simulink model "Xango_car_metamodel_V1_funcional"  (R2015a)
settings: Solver=ode45  StartTime=0  StopTime=6  FixedStep=1e-3  MaxStep=0.0001  RelTol=1e-19
values from neighbouring files (symbols this model uses):
  B_x_dd = C_s_dd / (C_x * D_dd)    [Xango_car_metamodel_SCRIPT.m]
  B_x_de = C_s_de / (C_x * D_de)    [Xango_car_metamodel_SCRIPT.m]
  B_x_td = C_s_td / (C_x * D_td)    [Xango_car_metamodel_SCRIPT.m]
  B_x_te = C_s_te / (C_x * D_te)    [Xango_car_metamodel_SCRIPT.m]
  B_y_dd = C_s_dd / (C_y * D_dd)    [Xango_car_metamodel_SCRIPT.m]
  B_y_de = C_s_de / (C_y * D_de)    [Xango_car_metamodel_SCRIPT.m]
  B_y_td = C_s_td / (C_y * D_td)    [Xango_car_metamodel_SCRIPT.m]
  B_y_te = C_s_te / (C_y * D_te)    [Xango_car_metamodel_SCRIPT.m]
  C_alpha_d = 0.5    [Xango_car_metamodel_SCRIPT.m]
  C_alpha_e = 0.5    [Xango_car_metamodel_SCRIPT.m]
  C_x = 1.0    (= 1)    [Xango_car_metamodel_SCRIPT.m]
  C_y = 1.627    [Xango_car_metamodel_SCRIPT.m]
  Cdd = 3e3    (= 3000)    [Xango_car_metamodel_SCRIPT.m]
  Cde = 3e3    (= 3000)    [Xango_car_metamodel_SCRIPT.m]
  Ctd = 5e3    (= 5000)    [Xango_car_metamodel_SCRIPT.m]
  Cte = 5e3    (= 5000)    [Xango_car_metamodel_SCRIPT.m]
  D_dd = mu * F_zdd    (= 1066.8375)    [Xango_car_metamodel_SCRIPT.m]
  D_de = mu * F_zde    (= 1066.8375)    [Xango_car_metamodel_SCRIPT.m]
  D_td = mu * F_ztd    (= 1066.8375)    [Xango_car_metamodel_SCRIPT.m]
  D_te = mu * F_zte    (= 1066.8375)    [Xango_car_metamodel_SCRIPT.m]
  E = 0.3336564873588197    (= 0.333656487359)    [Xango_car_metamodel_SCRIPT.m]
  H_cg = 0.3    [Xango_car_metamodel_SCRIPT.m]
  I_beta = 1e7    (= 10000000)    [Xango_car_metamodel_SCRIPT.m]
  I_p = 1.0    (= 1)    [Xango_car_metamodel_SCRIPT.m]
  I_psi = 1e7    (= 10000000)    [Xango_car_metamodel_SCRIPT.m]
  I_rho = 1e7    (= 10000000)    [Xango_car_metamodel_SCRIPT.m]
  If = 5e6    (= 5000000)    [Xango_car_metamodel_SCRIPT.m]
  It = 5e6    (= 5000000)    [Xango_car_metamodel_SCRIPT.m]
  Kdd = 3e6    (= 3000000)    [Xango_car_metamodel_SCRIPT.m]
  Kde = 3e6    (= 3000000)    [Xango_car_metamodel_SCRIPT.m]
  Kf = 3.01e7    (= 30100000)    [Xango_car_metamodel_SCRIPT.m]
  Kpdd = 2e6    (= 2000000)    [Xango_car_metamodel_SCRIPT.m]
  Kpde = 2e6    (= 2000000)    [Xango_car_metamodel_SCRIPT.m]
  Kptd = 2e6    (= 2000000)    [Xango_car_metamodel_SCRIPT.m]
  Kpte = 2e6    (= 2000000)    [Xango_car_metamodel_SCRIPT.m]
  Kt = 1.6e7    (= 16000000)    [Xango_car_metamodel_SCRIPT.m]
  Ktd = 5e6    (= 5000000)    [Xango_car_metamodel_SCRIPT.m]
  Kte = 5e6    (= 5000000)    [Xango_car_metamodel_SCRIPT.m]
  Ld = 1.2    [Xango_car_metamodel_SCRIPT.m]
  Lt = 1.2    [Xango_car_metamodel_SCRIPT.m]
  Mc = 300    [Xango_car_metamodel_SCRIPT.m]
  Msd = 100    [Xango_car_metamodel_SCRIPT.m]
  Mst = 120    [Xango_car_metamodel_SCRIPT.m]
  Rdp = 0.3    [Xango_car_metamodel_SCRIPT.m]
  tau_F = 500    [Xango_car_metamodel_SCRIPT.m]
  tau_M = 1000    [Xango_car_metamodel_SCRIPT.m]
  W2 = 0.45    [Xango_car_metamodel_SCRIPT.m]
undefined symbols (not defined in the file or in its folder): Cphi, Ctheta
settings Model: SnapshotBufferSize=1  SnapshotInterval=1  CovModelRefEnable=off  Creator=Vergilio  LastModifiedBy=joao_
settings DataIOCC: LimitDataPoints=off  SaveFormat=Dataset
settings HardwareCC: ProdBitPerPointer=64  ProdLargestAtomicFloat=Float  ProdIntDivRoundTo=Zero  ProdEndianess=LittleEndian  ProdHWDeviceType=Specified
settings ModelReferenceCC: PropagateSignalLabelsOutOfModel=on

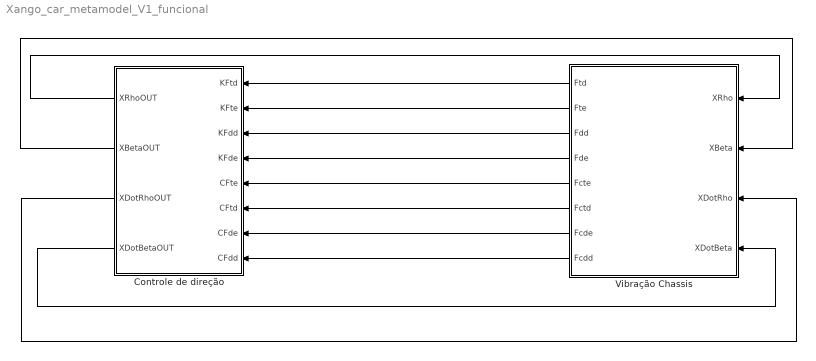
== system Xango_car_metamodel_V1_funcional ==
  "Controle de direção " : Subsystem
  Vibração Chassis : Subsystem
  wires:
  Vibração Chassis/1(Ftd) -> "Controle de direção "/1("KFtd ")
  Vibração Chassis/2(Fte) -> "Controle de direção "/2("KFte ")
  Vibração Chassis/3(Fdd) -> "Controle de direção "/3(KFdd)
  Vibração Chassis/4("Fde ") -> "Controle de direção "/4(KFde)
  Vibração Chassis/5(Fcte) -> "Controle de direção "/5("CFte ")
  Vibração Chassis/6(Fctd) -> "Controle de direção "/6("CFtd ")
  Vibração Chassis/7(Fcde) -> "Controle de direção "/7("CFde ")
  Vibração Chassis/8(Fcdd) -> "Controle de direção "/8("CFdd ")
  "Controle de direção "/1(XRhoOUT) -> Vibração Chassis/1(XRho)
  "Controle de direção "/2(XBetaOUT) -> Vibração Chassis/2(XBeta)
  "Controle de direção "/3("XDotRhoOUT ") -> Vibração Chassis/3(XDotRho)
  "Controle de direção "/4("XDotBetaOUT ") -> Vibração Chassis/4("XDotBeta ")

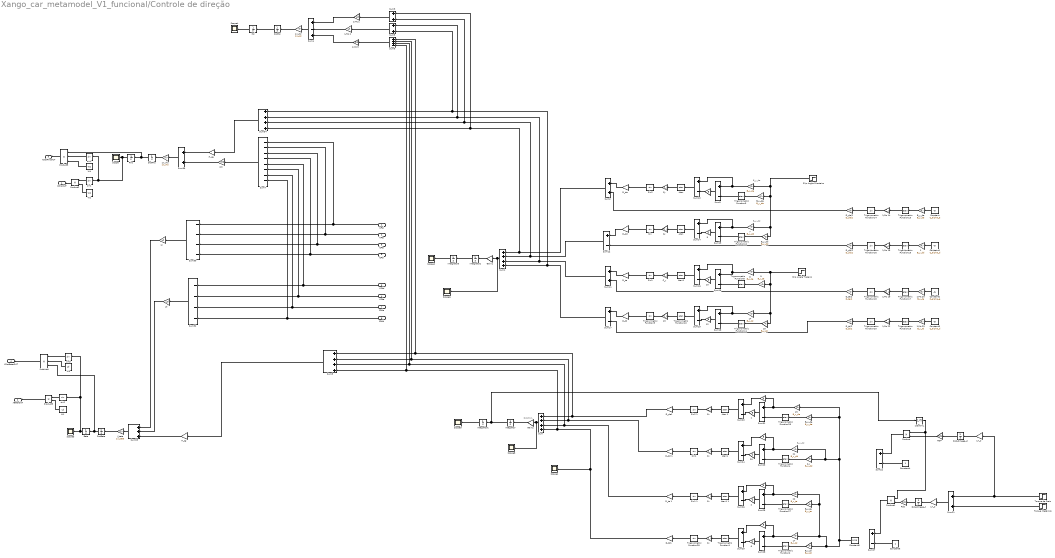
== system Xango_car_metamodel_V1_funcional/Controle de direção  ==
  note: DdotXVL
  note: B_y_de
  note: B_y_dd
  note: B_x_dd
  "KFtd " : Inport
  "KFte " : Inport  Port=2
  KFdd : Inport  Port=3
  KFde : Inport  Port=4
  "CFte " : Inport  Port=5
  "CFtd " : Inport  Port=6
  "CFde " : Inport  Port=7
  "CFdd " : Inport  Port=8
   {,1..2,5..6,10,12,20} (8 alike) : Gain  Gain=E
   {,,,} (4 alike) : Gain  Gain=9
   Cx{,,,} (4 alike) : Gain  Gain=C_x
  " 1/I_p" : Gain  Gain=1/I_p
  " 1/I_p " : Gain  Gain=1/I_p
  " 13" : Gain  Gain=C_y
  " 14" : Gain  Gain=B_y_td
  " 15" : Gain  Gain=B_y_td
  " 17" : Gain  Gain=B_x_td
  " 19" : Gain  Gain=B_x_de
  " 21" : Gain  Gain=B_x_dd
  " 22" : Gain  Gain=B_x_te
  " 24" : Gain  Gain=B_x_dd
  " 7" : Gain  Gain=B_y_dd
  " 8" : Gain  Gain=B_y_te
  " 9" : Gain  Gain=B_y_te
  " B_x_de " : Gain  Gain=B_x_de
  " B_x_td" : Gain  Gain=B_x_td
  " B_x_te" : Gain  Gain=B_x_te
  " C_y" : Gain  Gain=C_y
  " Cy" : Gain  Gain=C_y
  " Cy " : Gain  Gain=C_y
  " RDP" : Gain  Gain=Rdp
  " Rdp" : Gain  Gain=Rdp
  "       " : Gain  Gain=B_y_de
  " 1/I_rho " : Gain  Gain=1/I_rho
  " B_y_de" : Gain  Gain=B_y_de
  1 : Gain  Gain=B_y_dd
  1/DotXVL : Product  Inputs=/
  "1/I_Psi " : Gain  Gain=1/I_psi
  1/Mc 1 : Gain  Gain=Ld
  1/Mc {14,16,19,22} (4 alike) : Gain  Gain=C_y
  1/Mc 2 : Gain  Gain=Lt
  1/Mc 20 : Gain  Gain=B_y_te
  1/Mc 23 : Gain  Gain=B_y_td
  1/Mc 3 : Gain  Gain=W2
  Atan : Trigonometry  Operator=atan
  "Atan " : Trigonometry  Operator=atan
  Atan 1 : Trigonometry  Operator=atan
  Atan1 : Trigonometry  Operator=atan
  "Atan1 " : Trigonometry  Operator=atan
  Atan1 1 : Trigonometry  Operator=atan
  B_y_dd : Gain  Gain=B_y_dd
  B_y_de : Gain  Gain=B_y_de
  Beta : Integrator
  Constant : Constant  Value=C_alpha_e
  Constant1 : Constant  Value=C_alpha_d
  Constant2 : Constant  Value=C_alpha_e
  Constant3 : Constant  Value=C_alpha_d
  Constant4 : Constant
  Constant5 : Constant  Value=0.25
  Constant6 : Constant
  "D_dd " : Gain  Gain=D_dd
  D_dd 1 : Gain  Gain=D_dd
  D_dd/2 : Gain  Gain=D_dd/2
  D_de : Gain  Gain=D_de
  D_de/2 : Gain  Gain=D_de/2
  D_de1 : Gain  Gain=D_de
  D_td : Gain  Gain=D_td
  D_td/2 : Gain  Gain=D_td/2
  D_td1 : Gain  Gain=D_td
  "D_te " : Gain  Gain=D_te
  D_te 1 : Gain  Gain=D_te
  D_te/2 : Gain  Gain=D_te/2
  DotBeta : Integrator
  DotPsi : Integrator
  DotRho : Integrator
  Dot_Omega_d : Integrator
  Dot_Omega_t : Integrator
  Gain1 : Gain  Gain=1/Mc
  Gain2 : Gain  Gain=1/Mc
  "H_cg " : Gain  Gain=H_cg
  "H_cg   " : Gain  Gain=H_cg
  "I_beta " : Gain  Gain=1/I_beta
  Integrator : Integrator  InitialCondition=1
  Integrator1 : Integrator
  Integrator2 : Integrator
  Integrator3 : Integrator
  "Ld " : Gain  Gain=Ld
  "Lt " : Gain  Gain=Lt
  Product{,1..3} (4 alike) : Product
  Product4 : Product  Inputs=3
  Product5 : Product  Inputs=3
  Psi : Integrator
  Rho : Integrator
  Scope{,1..6,8} (8 alike) : Scope
      Scope settings: SaveName=ScopeData3
      Scope1 settings: YMin=-1000  YMax=1000  SaveName=ScopeData2
      Scope2 settings: SaveName=ScopeData9
      Scope3 settings: SaveName=ScopeData6
      Scope4 settings: TimeRange=4.999000000000002  YMin=1.8  YMax=2.2  SaveName=ScopeData7
      Scope5 settings: YMin=-11000  YMax=0  SaveName=ScopeData8
      Scope6 settings: YMin=0  YMax=65  SaveName=ScopeData4
      Scope8 settings: YMin=-3982.53  YMax=-3982.53  SaveName=ScopeData10
  Sin : Trigonometry
  Sin1 : Trigonometry
  "Sin1 " : Trigonometry
  Sin1 1 : Trigonometry
  "Sin2 " : Trigonometry
  Sin2 1 : Trigonometry
  "Slip Angle Dianteiro " : Step  Time=5  After=9  SampleTime=0
  "Slip Angle Traseiro " : Step  Time=5  SampleTime=0
  Sum{,1,8,34} (4 alike) : Sum  Inputs=++++
  Sum{9..10,12..20,22..29,31} (20 alike) : Sum  Inputs=+-
  Sum{2..3,5,11,21,35} (6 alike) : Sum
  Sum30 : Sum  Inputs=----
  Sum32 : Sum  Inputs=----
  Sum33 : Sum  Inputs=+++
  Sum4 : Sum  Inputs=+-+
  Sum6 : Sum  Inputs=+-+-
  Sum7 : Sum  Inputs=--------
  Torque Mecânico : Step  After=tau_M  SampleTime=0
  Torque de Freio : Step  Time=0  After=-tau_F  SampleTime=0
  Trigonometric Function{1..4,8,10..13,15,17,19,26..27} (14 alike) : Trigonometry  Operator=atan
  Trigonometric Function{9,14,16,18,20,28} (6 alike) : Trigonometry
  W1 : Constant  Value=Ld
  W2 : Constant  Value=W2
  "W2 " : Gain  Gain=W2
  W3 : Constant  Value=Ld
  W4 : Constant  Value=W2
  sin{1..4} (4 alike) : Trigonometry
  XRhoOUT : Outport
  XBetaOUT : Outport  Port=2
  "XDotRhoOUT " : Outport  Port=3
  "XDotBetaOUT " : Outport  Port=4
  wires:
  Sum3/1 -> 1/Mc 1/1
  Sum/1 -> Scope8/1, Gain2/1
  Integrator/1 -> 1/DotXVL/1, Integrator1/1  "DotXVL"
  1/Mc 3/1 -> Sum4/3
  Sum17/1 -> Sum1/4, Sum5/2, Sum34/1  "Fy_Td"
  Integrator2/1 -> Integrator3/1  "DotXVT"
  Integrator3/1 -> Scope2/1  "X_VT"
  Sum6/1 -> 1/Mc 3/1
  DotPsi/1 -> Psi/1
  Integrator1/1 -> Scope5/1  "X_VL"
  Sum4/1 -> "1/I_Psi "/1
  "1/I_Psi "/1 -> DotPsi/1
  Sum5/1 -> 1/Mc 2/1
  1/Mc 2/1 -> Sum4/2
  1/Mc 1/1 -> Sum4/1
  "H_cg   "/1 -> Sum35/1
  DotRho/1 -> Product5/1, Rho/1
  Rho/1 -> sin4/1, sin1/1, Scope/1
  Sum7/1 -> "W2 "/1
  " 1/I_rho "/1 -> DotRho/1
  DotBeta/1 -> Product4/3, Beta/1
  Beta/1 -> sin3/1, sin2/1, Scope3/1
  "H_cg "/1 -> Sum33/3
  "I_beta "/1 -> DotBeta/1
  Psi/1 -> Scope4/1
  Sum8/1 -> "H_cg "/1
  " C_y"/1 -> "Sin1 "/1
  "Sin1 "/1 -> "D_te "/1
  "Slip Angle Traseiro "/1 -> " 15"/1, " 14"/1, " 9"/1, " 8"/1
  " 8"/1 -> Sum16/1, Sum15/1
  Trigonometric Function8/1 -> Sum15/2
  " 9"/1 -> Trigonometric Function8/1
  Sum15/1 -> " 10"/1
  " 10"/1 -> Sum16/2
  Sum16/1 -> "Atan1 "/1
  "Atan1 "/1 -> " C_y"/1
  "D_te "/1 -> Sum11/1
  " Cy "/1 -> "Sin2 "/1
  "Sin2 "/1 -> D_de/1
  "Slip Angle Dianteiro "/1 -> " 7"/1, B_y_dd/1, " B_y_de"/1, "       "/1
  "       "/1 -> Sum10/1, Sum9/1
  Trigonometric Function3/1 -> Sum9/2
  " B_y_de"/1 -> Trigonometric Function3/1
  Sum9/1 -> " "/1
  " "/1 -> Sum10/2
  Sum10/1 -> "Atan "/1
  "Atan "/1 -> " Cy "/1
  D_de/1 -> Sum2/1
  " Cy"/1 -> Sin/1
  Sin/1 -> "D_dd "/1
  " 7"/1 -> Sum14/1, Sum13/1
  Trigonometric Function12/1 -> Sum13/2
  B_y_dd/1 -> Trigonometric Function12/1
  Sum13/1 -> " 5"/1
  " 5"/1 -> Sum14/2
  Sum14/1 -> Atan/1
  Atan/1 -> " Cy"/1
  "D_dd "/1 -> Sum12/1
  " 13"/1 -> Trigonometric Function9/1
  Trigonometric Function9/1 -> D_td/1
  " 14"/1 -> Sum19/1, Sum18/1
  Trigonometric Function11/1 -> Sum18/2
  " 15"/1 -> Trigonometric Function11/1
  Sum18/1 -> " 12"/1
  " 12"/1 -> Sum19/2
  Sum19/1 -> Trigonometric Function10/1
  Trigonometric Function10/1 -> " 13"/1
  D_td/1 -> Sum17/1
  D_dd/2/1 -> Sum12/2
  D_te/2/1 -> Sum11/2
  D_td/2/1 -> Sum17/2
  Trigonometric Function14/1 -> D_de/2/1
  1/Mc 14/1 -> Trigonometric Function14/1
  Trigonometric Function13/1 -> 1/Mc 14/1
  B_y_de/1 -> Trigonometric Function13/1
  Constant/1 -> B_y_de/1
  D_de/2/1 -> Sum2/2
  1/Mc 16/1 -> Trigonometric Function16/1
  Trigonometric Function15/1 -> 1/Mc 16/1
  1/1 -> Trigonometric Function15/1
  Constant1/1 -> 1/1
  Trigonometric Function18/1 -> D_te/2/1
  1/Mc 19/1 -> Trigonometric Function18/1
  Trigonometric Function17/1 -> 1/Mc 19/1
  1/Mc 20/1 -> Trigonometric Function17/1
  Constant2/1 -> 1/Mc 20/1
  Trigonometric Function20/1 -> D_td/2/1
  1/Mc 22/1 -> Trigonometric Function20/1
  Trigonometric Function19/1 -> 1/Mc 22/1
  1/Mc 23/1 -> Trigonometric Function19/1
  Constant3/1 -> 1/Mc 23/1
  Trigonometric Function16/1 -> D_dd/2/1
  Sum2/1 -> Sum1/1, Sum3/1, Sum34/4  "Fy_De"
  Sum12/1 -> Sum1/2, Sum3/2, Sum34/3  "Fy_Dd"
  Sum11/1 -> Sum1/3, Sum5/1, Sum34/2  "Fy_Te"
  Gain1/1 -> Integrator2/1
  " Cx"/1 -> Sin1 1/1
  Sin1 1/1 -> D_te 1/1
  Trigonometric Function27/1 -> Sum25/2
  " B_x_te"/1 -> Trigonometric Function27/1
  Sum25/1 -> " 2"/1
  " 2"/1 -> Sum26/2
  Sum26/1 -> Atan1 1/1
  Atan1 1/1 -> " Cx"/1
  " Cx"/1 -> Sin2 1/1
  Sin2 1/1 -> D_de1/1
  " 19"/1 -> " "/1, Sum31/1
  Trigonometric Function26/1 -> Sum31/2
  " B_x_de "/1 -> Trigonometric Function26/1
  Sum31/1 -> " 1"/1
  " 1"/1 -> Sum20/2
  Sum20/1 -> Atan 1/1
  Atan 1/1 -> " Cx"/1
  " Cx"/1 -> Sin1/1
  Sin1/1 -> D_dd 1/1
  Trigonometric Function4/1 -> Sum23/2
  " 24"/1 -> Trigonometric Function4/1
  Sum23/1 -> " 20"/1
  " 20"/1 -> Sum24/2
  Sum24/1 -> Atan1/1
  Atan1/1 -> " Cx"/1
  " Cx"/1 -> Trigonometric Function28/1
  Trigonometric Function28/1 -> D_td1/1
  Trigonometric Function2/1 -> Sum28/2
  " B_x_td"/1 -> Trigonometric Function2/1
  Sum28/1 -> " 6"/1
  " 6"/1 -> Sum29/2
  Sum29/1 -> Trigonometric Function1/1
  Trigonometric Function1/1 -> " Cx"/1
  D_de1/1 -> Sum8/1, Sum6/1, Sum/1  "Fx_De"
  D_dd 1/1 -> Sum8/2, Sum6/2, Sum/2  "Fx_Dd"
  D_te 1/1 -> Sum/3, Sum8/3, Sum6/3  "Fx_Te"
  D_td1/1 -> Scope1/1, Sum/4, Sum8/4, Sum6/4  "Fx_Td"
  Gain2/1 -> Integrator/1
  " "/1 -> Sum20/1
  " 21"/1 -> " "/1, Sum23/1
  " "/1 -> Sum24/1
  " 22"/1 -> " "/1, Sum25/1
  " "/1 -> Sum26/1
  " 17"/1 -> " "/1, Sum28/1
  " "/1 -> Sum29/1
  Torque Mecânico/1 -> Sum21/2
  " 1/I_p "/1 -> Dot_Omega_d/1
  Constant4/1 -> Sum22/2
  Dot_Omega_d/1 -> " RDP"/1
  " RDP"/1 -> Product/2
  Product/1 -> Sum22/1
  Torque de Freio/1 -> Sum21/1, " 1/I_p "/1
  Sum1/1 -> Scope6/1, Gain1/1
  Sum21/1 -> " 1/I_p"/1
  " 1/I_p"/1 -> Dot_Omega_t/1
  1/DotXVL/1 -> Product1/1, Product/1
  Dot_Omega_t/1 -> " Rdp"/1
  " Rdp"/1 -> Product1/2
  Product1/1 -> Sum27/1
  "KFtd "/1 -> Sum30/1, Sum7/1
  KFdd/1 -> Sum32/1, Sum7/5
  "KFte "/1 -> Sum30/2, Sum7/2
  KFde/1 -> Sum32/2, Sum7/6
  "CFte "/1 -> Sum30/3, Sum7/3
  "CFtd "/1 -> Sum30/4, Sum7/4
  "CFde "/1 -> Sum7/7, Sum32/3
  "CFdd "/1 -> Sum7/8, Sum32/4
  sin1/1 -> Product2/1
  W2/1 -> Product2/2
  Product2/1 -> XRhoOUT/1
  sin2/1 -> Product3/1
  W1/1 -> Product3/2
  Product3/1 -> XBetaOUT/1
  sin3/1 -> Product4/1
  W3/1 -> Product4/2
  W4/1 -> Product5/3
  sin4/1 -> Product5/2
  Product5/1 -> "XDotRhoOUT "/1
  Product4/1 -> "XDotBetaOUT "/1
  Sum30/1 -> "Lt "/1
  Sum32/1 -> "Ld "/1
  Sum33/1 -> "I_beta "/1
  "Ld "/1 -> Sum33/2
  "Lt "/1 -> Sum33/1
  Sum34/1 -> "H_cg   "/1
  Sum35/1 -> " 1/I_rho "/1
  "W2 "/1 -> Sum35/2
  Constant5/1 -> " B_x_td"/1, " 22"/1, " B_x_te"/1, " 17"/1, " 19"/1, " B_x_de "/1, " 21"/1, " 24"/1
  Constant6/1 -> Sum27/2

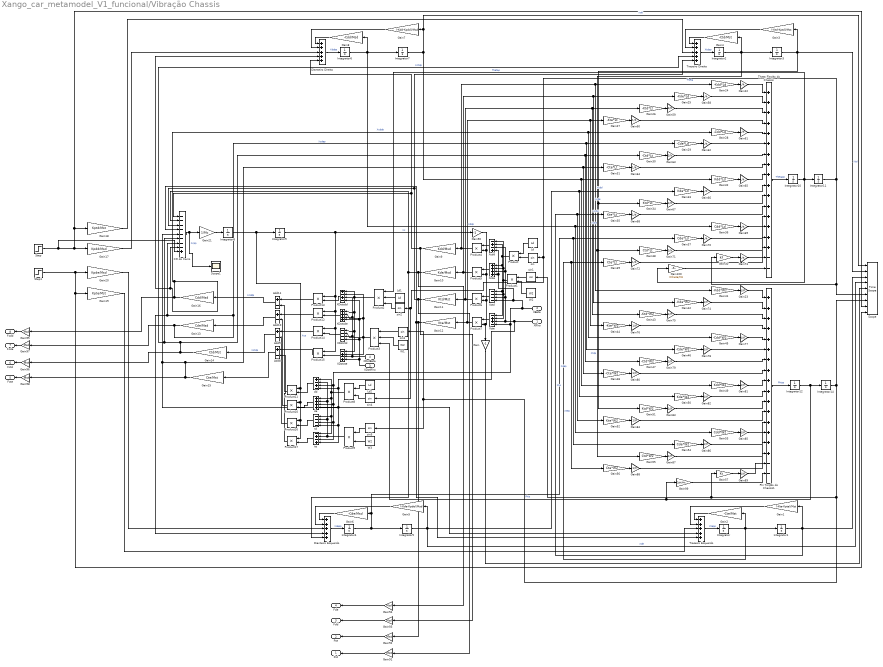
== system Xango_car_metamodel_V1_funcional/Vibração Chassis ==
  XRho : Inport
  XBeta : Inport  Port=2
  XDotRho : Inport  Port=3
  "XDotBeta " : Inport  Port=4
  Add{8..11} (4 alike) : Sum  Inputs=+-
  CG do Carro : Sum  Inputs=--------+
  Dianteiro Direito : Sum  Inputs=+++++
  Dianteiro Esquerdo : Sum  Inputs=+++++
  Gain : Gain  Gain=-1
  Gain1 : Gain  Gain=(-Kte-Kpte)/Mst
  Gain10 : Gain  Gain=Kde/Msd
  Gain100 : Gain  Gain=Ctheta/Mc
  Gain11 : Gain  Gain=Ktd/Mst
  Gain12 : Gain  Gain=Kte/Mst
  Gain13 : Gain  Gain=Cde/Msd
  Gain14 : Gain  Gain=Ctd/Mst
  Gain15 : Gain  Gain=Cte/Mst
  Gain16 : Gain  Gain=Cdd/Msd
  Gain17 : Gain  Gain=Kpdd/Msd
  Gain18 : Gain  Gain=Kptd/Mst
  Gain19 : Gain  Gain=Kpte/Mst
  Gain2 : Gain  Gain=-Cte/Mst
  Gain20 : Gain  Gain=Kpde/Msd
  Gain21 : Gain  Gain=1/Mc
  Gain{22,58..73} (17 alike) : Gain  Gain=1/It
  Gain{23,74..89} (17 alike) : Gain  Gain=1/If
  Gain24 : Gain  Gain=-Kdd*Ld
  Gain25 : Gain  Gain=-Kde*Ld
  Gain26 : Gain  Gain=-Ktd*Lt
  Gain27 : Gain  Gain=-Kte*Lt
  Gain28 : Gain  Gain=-Cdd*Ld
  Gain29 : Gain  Gain=-Cde*Ld
  Gain3 : Gain  Gain=(-Ktd-Kptd)/Mst
  Gain30 : Gain  Gain=-Ctd*Lt
  Gain31 : Gain  Gain=-Cte*Lt
  Gain32 : Gain  Gain=Kdd*Ld
  Gain33 : Gain  Gain=Kde*Ld
  Gain34 : Gain  Gain=Ktd*Lt
  Gain35 : Gain  Gain=Kte*Lt
  Gain36 : Gain  Gain=Cdd*Ld
  Gain37 : Gain  Gain=Cde*Ld
  Gain38 : Gain  Gain=Ctd*Lt
  Gain39 : Gain  Gain=Cte*Lt
  Gain4 : Gain  Gain=-Ctd/Mst
  Gain40 : Gain  Gain=Kf
  Gain41 : Gain  Gain=-Kdd*W2
  Gain42 : Gain  Gain=-Kde*W2
  Gain43 : Gain  Gain=-Ktd*W2
  Gain44 : Gain  Gain=-Kte*W2
  Gain45 : Gain  Gain=-Cdd*W2
  Gain46 : Gain  Gain=-Cde*W2
  Gain47 : Gain  Gain=-Ctd*W2
  Gain48 : Gain  Gain=-Cte*W2
  Gain49 : Gain  Gain=Kdd*W2
  Gain5 : Gain  Gain=(-Kde-Kpde)/Msd
  Gain50 : Gain  Gain=Kde*W2
  Gain51 : Gain  Gain=Ktd*W2
  Gain52 : Gain  Gain=Kte*W2
  Gain53 : Gain  Gain=Cdd*W2
  Gain54 : Gain  Gain=Cde*W2
  Gain55 : Gain  Gain=Ctd*W2
  Gain56 : Gain  Gain=Cte*W2
  Gain57 : Gain  Gain=Kt
  Gain6 : Gain  Gain=-Cde/Msd
  Gain7 : Gain  Gain=(-Kdd-Kpdd)/Msd
  Gain8 : Gain  Gain=-Cdd/Msd
  Gain9 : Gain  Gain=Kdd/Msd
  Gain90 : Gain  Gain=-1
  Gain{91..92,96,98} (4 alike) : Gain  Gain=Mst
  Gain{93..95,97} (4 alike) : Gain  Gain=Msd
  Gain99 : Gain  Gain=Cphi/Mc
  Integrator{,1..12} (13 alike) : Integrator
  Integrator14 : Integrator  UpperSaturationLimit=0.45  LowerSaturationLimit=-0.45
  Ld : Constant  Value=Ld
  Ld1 : Constant  Value=Ld
  Ld2 : Constant  Value=Ld
  Phi Torção do Chassis1 : Sum  Inputs=++++++++++++++++--
  Product{,1,4..17} (16 alike) : Product
  Product2 : Product  Inputs=3
  Product3 : Product  Inputs=3
  Scope : TimeScope  NumInputPorts=9
  Scope1 : Scope
  Step : Step  SampleTime=0
  Step1 : Step  Time=5  After=2  SampleTime=0
  Theta Flexão do Chassis : Sum  Inputs=++++++++++++++++--
  Traseiro Direito : Sum  Inputs=+++++
  Traseiro Esquerdo : Sum  Inputs=+++++
  W1 : Constant  Value=W2
  W2 : Constant  Value=W2
  W3 : Constant  Value=W2
  XDotcdd : Sum  Inputs=+-+-
  XDotcde : Sum  Inputs=++++
  XDotctd : Sum  Inputs=----
  XDotcte : Sum  Inputs=-+-+
  Xcdd : Sum  Inputs=-+-+
  Xcde : Sum  Inputs=++++
  Xctd : Sum  Inputs=----
  Xcte : Sum  Inputs=-++-
  dd : Sum  Inputs=+-+-
  de : Sum  Inputs=++++
  sin{,1..5} (6 alike) : Trigonometry
  td : Sum  Inputs=----
  te : Sum  Inputs=-+-+
  Ftd : Outport
  Fte : Outport  Port=2
  Fdd : Outport  Port=3
  "Fde " : Outport  Port=4
  Fcte : Outport  Port=5
  Fctd : Outport  Port=6
  Fcde : Outport  Port=7
  Fcdd : Outport  Port=8
  wires:
  Integrator1/1 -> Scope/3, Gain1/1, Gain52/1, Gain35/1  "Xte"
  Traseiro Esquerdo/1 -> Integrator/1  "Xtepp"
  Dianteiro Esquerdo/1 -> Integrator4/1  "Xdepp"
  Xcdd/1 -> Product4/1
  Gain9/1 -> Gain93/1, CG do Carro/1, Dianteiro Direito/5
  Integrator/1 -> Gain2/1, Gain56/1, Gain39/1, Integrator1/1  "Xtep"
  Xcde/1 -> Product5/1
  sin1/1 -> Product1/1
  Integrator8/1 -> Product17/1, Product16/1, Product10/1, Product11/1, Integrator9/1  "Xcp"
  Integrator2/1 -> Gain4/1, Gain38/1, Gain55/1, Integrator3/1  "Xtdp"
  Integrator14/1 -> Gain57/1, sin1/1, sin3/1, sin5/1, Scope/7
  Gain6/1 -> Dianteiro Esquerdo/1
  Dianteiro Direito/1 -> Integrator6/1  "Xddpp"
  Integrator11/1 -> Gain40/1, Scope/6, sin4/1, sin2/1, sin/1  "Theta"
  Integrator5/1 -> Scope/4, Gain5/1, Gain50/1, Gain33/1  "Xde"
  Gain5/1 -> Dianteiro Esquerdo/2
  Traseiro Direito/1 -> Integrator2/1  "Xtdpp"
  Gain8/1 -> Dianteiro Direito/1
  Gain7/1 -> Dianteiro Direito/2
  Gain3/1 -> Traseiro Direito/2
  Integrator10/1 -> Gain100/1, Product2/1, Integrator11/1  "Thetap"
  Gain1/1 -> Traseiro Esquerdo/2
  Integrator4/1 -> Integrator5/1, Gain54/1, Gain37/1, Gain6/1  "Xdep"
  Integrator12/1 -> Integrator14/1, Gain99/1, Product3/3  "Phip"
  Integrator9/1 -> Gain90/1, Product14/1, Product15/1, Product12/1, Product13/1  "Xc"
  sin/1 -> Product/2
  Gain2/1 -> Traseiro Esquerdo/1
  Integrator6/1 -> Gain8/1, Gain53/1, Gain36/1, Integrator7/1  "Xddp"
  W2/1 -> Product1/2
  Product/1 -> Xcdd/2, Xcte/1, Xctd/1, Xcde/1
  Integrator7/1 -> Gain7/1, Scope/1, Gain49/1, Gain32/1  "Xdd"
  Integrator3/1 -> Gain3/1, Gain34/1, Gain51/1, Scope/2  "Xtd"
  Gain4/1 -> Traseiro Direito/1
  Gain24/1 -> Gain22/1
  Gain10/1 -> Gain94/1, CG do Carro/2, Dianteiro Esquerdo/5
  Gain19/1 -> Traseiro Esquerdo/3
  CG do Carro/1 -> Scope1/1, Gain21/1  "Xcpp"
  Gain15/1 -> Gain98/1, Gain31/1, Gain48/1, CG do Carro/5, Traseiro Esquerdo/4
  sin3/1 -> Product3/1
  Gain22/1 -> Theta Flexão do Chassis/1
  W1/1 -> Product3/2
  Xctd/1 -> Product6/1
  Gain18/1 -> Traseiro Direito/3
  Step1/1 -> Scope/9, Gain19/1, Gain20/1
  sin2/1 -> Product2/3
  Step/1 -> CG do Carro/9, Scope/8, Gain18/1, Gain17/1
  Product4/1 -> Gain41/1, Gain24/1, Gain9/1  "Xcdd"
  Product6/1 -> Gain43/1, Gain26/1, Gain11/1  "Xctd"
  Xcte/1 -> Product7/1
  Gain12/1 -> Traseiro Esquerdo/5, CG do Carro/4, Gain92/1
  Gain11/1 -> Gain91/1, Traseiro Direito/5, CG do Carro/3
  Phi Torção do Chassis1/1 -> Integrator12/1  "Phipp"
  Product1/1 -> Xcte/2, Xctd/2, Xcdd/1, Xcde/2
  Product7/1 -> Gain44/1, Gain27/1, Gain12/1  "Xcte"
  Gain16/1 -> CG do Carro/8, Dianteiro Direito/4, Gain45/1, Gain28/1, Gain95/1  "Xcddp"
  Gain20/1 -> Dianteiro Esquerdo/3
  Gain21/1 -> Integrator8/1
  Gain13/1 -> Gain97/1, CG do Carro/7, Dianteiro Esquerdo/4, Gain46/1, Gain29/1  "Xcdep"
  Product5/1 -> Gain42/1, Gain25/1, Gain10/1  "Xcde"
  Gain14/1 -> Gain96/1, Gain47/1, Gain30/1, CG do Carro/6, Traseiro Direito/4  "Xctdp"
  Ld1/1 -> Product2/2
  Theta Flexão do Chassis/1 -> Integrator10/1  "Thetapp"
  Gain17/1 -> Dianteiro Direito/3
  Gain58/1 -> Theta Flexão do Chassis/2
  Gain26/1 -> Gain59/1
  Gain72/1 -> Theta Flexão do Chassis/16
  Gain40/1 -> Gain73/1
  Gain33/1 -> Gain66/1
  Gain34/1 -> Gain67/1
  Gain37/1 -> Gain70/1
  Gain73/1 -> Theta Flexão do Chassis/17
  Gain35/1 -> Gain68/1
  Gain66/1 -> Theta Flexão do Chassis/10
  Gain30/1 -> Gain63/1
  Gain60/1 -> Theta Flexão do Chassis/4
  Gain29/1 -> Gain62/1
  Gain64/1 -> Theta Flexão do Chassis/8
  Gain32/1 -> Gain65/1
  Gain25/1 -> Gain58/1
  Gain65/1 -> Theta Flexão do Chassis/9
  Gain59/1 -> Theta Flexão do Chassis/3
  Gain68/1 -> Theta Flexão do Chassis/12
  Gain36/1 -> Gain69/1
  Gain27/1 -> Gain60/1
  Gain61/1 -> Theta Flexão do Chassis/5
  Gain69/1 -> Theta Flexão do Chassis/13
  Gain62/1 -> Theta Flexão do Chassis/6
  Gain63/1 -> Theta Flexão do Chassis/7
  Gain31/1 -> Gain64/1
  Gain38/1 -> Gain71/1
  Gain67/1 -> Theta Flexão do Chassis/11
  Gain70/1 -> Theta Flexão do Chassis/14
  Gain71/1 -> Theta Flexão do Chassis/15
  Gain39/1 -> Gain72/1
  Gain28/1 -> Gain61/1
  Gain54/1 -> Gain86/1
  Gain74/1 -> Phi Torção do Chassis1/2
  Gain83/1 -> Phi Torção do Chassis1/11
  Gain43/1 -> Gain75/1
  Gain78/1 -> Phi Torção do Chassis1/6
  Gain82/1 -> Phi Torção do Chassis1/10
  Gain84/1 -> Phi Torção do Chassis1/12
  Gain75/1 -> Phi Torção do Chassis1/3
  Gain45/1 -> Gain77/1
  Gain79/1 -> Phi Torção do Chassis1/7
  Gain86/1 -> Phi Torção do Chassis1/14
  Gain49/1 -> Gain81/1
  Gain50/1 -> Gain82/1
  Gain44/1 -> Gain76/1
  Gain52/1 -> Gain84/1
  Gain77/1 -> Phi Torção do Chassis1/5
  Gain55/1 -> Gain87/1
  Gain87/1 -> Phi Torção do Chassis1/15
  Gain47/1 -> Gain79/1
  Gain51/1 -> Gain83/1
  Gain56/1 -> Gain88/1
  Gain88/1 -> Phi Torção do Chassis1/16
  Gain76/1 -> Phi Torção do Chassis1/4
  Gain41/1 -> Gain23/1
  Gain80/1 -> Phi Torção do Chassis1/8
  Gain81/1 -> Phi Torção do Chassis1/9
  Gain42/1 -> Gain74/1
  Gain23/1 -> Phi Torção do Chassis1/1
  Gain46/1 -> Gain78/1
  Gain48/1 -> Gain80/1
  Gain85/1 -> Phi Torção do Chassis1/13
  Gain53/1 -> Gain85/1
  W3/1 -> Product9/2
  td/1 -> Product16/2
  te/1 -> Product17/2
  Ld/1 -> Product/1
  sin5/1 -> Product9/1
  Product16/1 -> Add9/2
  Add8/1 -> Gain15/1
  Add9/1 -> Gain14/1  "Xctdp"
  Gain89/1 -> Phi Torção do Chassis1/17
  XDotctd/1 -> Product14/2
  Ld2/1 -> Product8/1
  Product15/1 -> Add8/1
  Gain90/1 -> Product4/2, Product5/2, Product6/2, Product7/2, Gain/1
  de/1 -> Product10/2
  Product17/1 -> Add8/2
  Product10/1 -> Add10/2
  Product14/1 -> Add9/1
  Add10/1 -> Gain13/1
  XDotcdd/1 -> Product13/2
  Product12/1 -> Add10/1
  Product2/1 -> XDotcdd/1, XDotcte/1, XDotctd/1, XDotcde/1
  Product13/1 -> Add11/1
  Product9/1 -> te/2, td/2, de/2, dd/2
  Gain/1 -> Scope/5
  XDotcde/1 -> Product12/2
  Product11/1 -> Add11/2
  XDotcte/1 -> Product15/2
  dd/1 -> Product11/2
  Gain57/1 -> Gain89/1
  Product3/1 -> XDotcdd/2, XDotcde/2, XDotctd/2, XDotcte/2
  sin4/1 -> Product8/2
  Product8/1 -> te/1, td/1, de/1, dd/1
  Add11/1 -> Gain16/1  "Xcddp"
  Gain94/1 -> "Fde "/1
  Gain93/1 -> Fdd/1
  Gain92/1 -> Fte/1
  Gain91/1 -> Ftd/1
  Gain95/1 -> Fcdd/1
  Gain97/1 -> Fcde/1
  Gain98/1 -> Fcte/1
  Gain96/1 -> Fctd/1
  XRho/1 -> de/4, te/4, td/4, dd/4, Xcdd/3, Xcde/3, Xctd/3, Xcte/3
  XBeta/1 -> te/3, td/3, de/3, dd/3, Xcte/4, Xctd/4, Xcdd/4, Xcde/4
  "XDotBeta "/1 -> XDotcte/3, XDotcdd/3, XDotcde/3, XDotctd/3
  XDotRho/1 -> XDotcte/4, XDotctd/4, XDotcdd/4, XDotcde/4
  Gain99/1 -> Phi Torção do Chassis1/18
  Gain100/1 -> Theta Flexão do Chassis/18
